simulink model "Climb"  (R2025b)
settings: Solver=VariableStepAuto  StartTime=0.0  StopTime=40  RelTol=1e-3  AbsTol=1e-3  EnableMultiTasking=on
undefined symbols (not defined in the file): X, Y, Z
libraries: sm_lib x52, nesl_utility x15
(part 2 of 2)

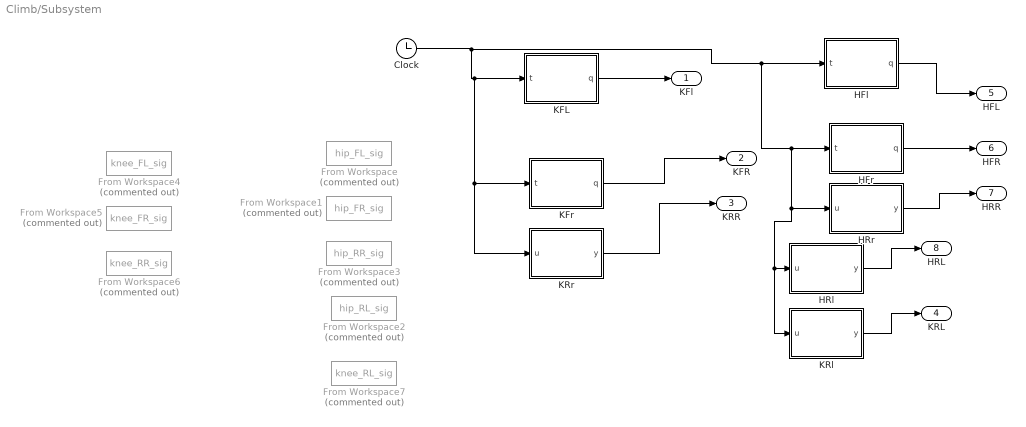
== system Climb/Subsystem ==
  Clock : Clock
  From Workspace : FromWorkspace  Commented=on  VariableName=hip_FL_sig
  From Workspace1 : FromWorkspace  Commented=on  VariableName=hip_FR_sig
  From Workspace2 : FromWorkspace  Commented=on  VariableName=hip_RL_sig
  From Workspace3 : FromWorkspace  Commented=on  VariableName=hip_RR_sig
  From Workspace4 : FromWorkspace  Commented=on  VariableName=knee_FL_sig
  From Workspace5 : FromWorkspace  Commented=on  VariableName=knee_FR_sig
  From Workspace6 : FromWorkspace  Commented=on  VariableName=knee_RR_sig
  From Workspace7 : FromWorkspace  Commented=on  VariableName=knee_RL_sig
  HFl : MATLAB Function  TreatAsAtomicUnit=on
  HFr : MATLAB Function  TreatAsAtomicUnit=on
  HRl : MATLAB Function  TreatAsAtomicUnit=on
  HRr : MATLAB Function  TreatAsAtomicUnit=on
  KFL : MATLAB Function  TreatAsAtomicUnit=on
  KFr : MATLAB Function  TreatAsAtomicUnit=on
  KRl : MATLAB Function  TreatAsAtomicUnit=on
  KRr : MATLAB Function  TreatAsAtomicUnit=on
  KFl : Outport
  KFR : Outport  Port=2
  KRR : Outport  Port=3
  KRL : Outport  Port=4
  HFL : Outport  Port=5
  HFR : Outport  Port=6
  HRR : Outport  Port=7
  HRL : Outport  Port=8
  wires:
  KFL/1(q) -> KFl/1
  KFr/1(q) -> KFR/1
  KRr/1(y) -> KRR/1
  HFl/1(q) -> HFL/1
  HFr/1(q) -> HFR/1
  HRr/1(y) -> HRR/1
  HRl/1(y) -> HRL/1
  KRl/1(y) -> KRL/1
  Clock/1 -> KRl/1(u), HRl/1(u), HRr/1(u), HFr/1(t), HFl/1(t), KRr/1(u), KFr/1(t), KFL/1(t)

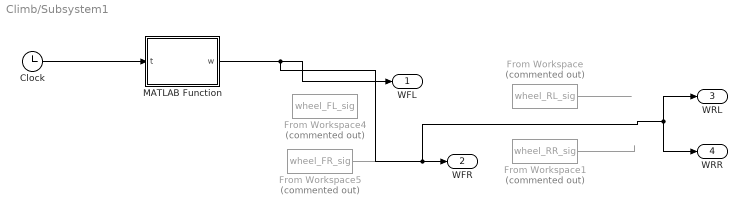
== system Climb/Subsystem1 ==
  Clock : Clock
  From Workspace : FromWorkspace  Commented=on  VariableName=wheel_RL_sig
  From Workspace1 : FromWorkspace  Commented=on  VariableName=wheel_RR_sig
  From Workspace4 : FromWorkspace  Commented=on  VariableName=wheel_FL_sig
  From Workspace5 : FromWorkspace  Commented=on  VariableName=wheel_FR_sig
  MATLAB Function : MATLAB Function  TreatAsAtomicUnit=on
  WFL : Outport
  WFR : Outport  Port=2
  WRL : Outport  Port=3
  WRR : Outport  Port=4
  wires:
  From Workspace/1 -> ?
  From Workspace5/1 -> ?
  From Workspace1/1 -> ?
  MATLAB Function/1(w) -> WRR/1, WRL/1, WFR/1, WFL/1
  Clock/1 -> MATLAB Function/1(t)

== matlab function Climb/Subsystem1/MATLAB Function ==
  data: t input; w output
function w = wheel_speed(t)
%#codegen
if t < 3
    w = 0;           % wait while FL lifts
elseif t < 6
    w = -0.2*t;        % slow forward
elseif t < 8
    w = 0;           % stop while FR lifts
elseif t < 26
    w = -0.2*t;        % move forward with FR lifted
else
    w = -0.2*t;           % stop when both straighten
end
end

== matlab function Climb/Subsystem/KFr ==
  data: t input; q output
function q = knee_FR_motion(t)
%#codegen
if t < 6
    q = 0;                          % wait
elseif t < 8
    q = -deg2rad(60) * (t - 6)/2;  % bend opposite to tuck while lifting
elseif t < 20
    q = -deg2rad(60);               % hold bend while moving
else
    q = -deg2rad(60);
end
end

== matlab function Climb/Subsystem/KRr ==
  data: u input; y output
function y = fcn(u)

y = 0;

== matlab function Climb/Subsystem/HFl ==
  data: t input; q output
function q = hip_FL_motion(t)
%#codegen
if t < 1
    q = 0;                       % neutral
elseif t < 3
    q = deg2rad(60) * (t - 1)/2;  % lift hip slowly 1→3s
elseif t < 20
    q = deg2rad(60);             % hold while moving forward 3→13s
elseif t < 25
    q = deg2rad(60) + (deg2rad(90) - deg2rad(60)) * (t - 20) / (5);
else
    q = deg2rad(90);                       % neutral
end
end

== matlab function Climb/Subsystem/HFr ==
  data: t input; q output
function q = hip_FR_motion(t)
%#codegen
if t < 6
    q = 0;                        % wait until FL is mostly on step
elseif t < 8
    q = deg2rad(90) * (t - 6)/2;   % lift FR slowly
elseif t < 20
    q = deg2rad(90);               % hold while moving forward
% elseif t < 100
%     q = deg2rad(90) * (100 - t)/2;  % straighten gradually
else
    q = deg2rad(90);
end
end

== matlab function Climb/Subsystem/HRr ==
  data: u input; y output
function y = fcn(u)

y = 0;

== matlab function Climb/Subsystem/HRl ==
  data: u input; y output
function y = fcn(u)

y = 0;

== matlab function Climb/Subsystem/KRl ==
  data: u input; y output
function y = fcn(u)

y = 0;

== matlab function Climb/Subsystem/KFL ==
  data: t input; q output
function q = knee_FL_motion(t)
%#codegen
if t < 1
    q = 0;
elseif t < 3
    q = deg2rad(25) * (t - 1)/2;   % bend knee slowly
elseif t < 20
    q = deg2rad(25);               % hold bend while moving
elseif t < 25
    q = deg2rad(25) - (deg2rad(25) + deg2rad(60)) * (t - 20) / (5);  % straighten gradually
else
    q = -deg2rad(60);
end
end
